simulink model "Kubon_lab10_3_sim"  (R2020b)
settings: Solver=VariableStepAuto  StartTime=0.0  StopTime=T_stop  RelTol=1e-3
values from neighbouring files (symbols this model uses):
  A = [ (-cpN*ppN*fk0-ks1-k0)/(Cv1) , k0/Cv1 ; (k0+cpN*ppN*fk0)/(Cv2) , (-k0-cpN*ppN*fk0-ks2)/(Cv2)  ]    [Kubon_lab10.m]    (also in Kubon_lab8.m = [-a1/A1 , a1/A1 ; a1/A2 , (-a1-a2)/A2])
  B = [(cpN*ppN*fk0)/(Cv1) , ks2/Cv1 ; 0 , ks2/Cv2 ]    [Kubon_lab10.m]    (also in Kubon_lab8.m = [1/A1 , 0 ; 0 , 1/A2])
  C = eye(2)    [Kubon_lab10.m]    (also in Kubon_lab8.m)
  D = zeros(2)    [Kubon_lab10.m]    (also in Kubon_lab8.m)
  dTkz = 2.0    (= 2)    [Kubon_lab10.m]    (also in Kubon_lab9.m = 0)
  dTzew = 0.0    (= 0)    [Kubon_lab10.m]    (also in Kubon_lab9.m)
  t0 = 50.0    (= 50)    [Kubon_lab10.m]    (also in Kubon_lab4.m = 5; Kubon_lab5.m = 0; Kubon_lab6.m = 5; Kubon_lab6_test.m = 0)
  Tkz0 = TkzN*0.7    (= 21)    [Kubon_lab10.m]    (also in Kubon_lab9.m = 30)
  Tw0_w = [Tw10,Tw20]    [Kubon_lab10.m]
  Tzew0 = TzewN    (= -20)    [Kubon_lab10.m]    (also in Kubon_lab9.m)
settings Model: Creator=pkubo  LastModifiedBy=pkubo

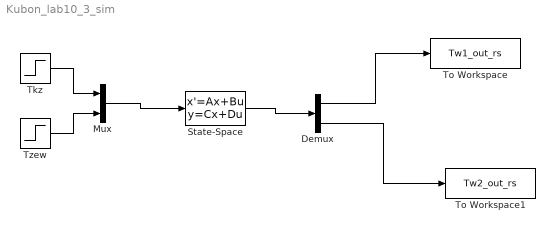
== system Kubon_lab10_3_sim ==
  Demux : Demux  Outputs=2
  Mux : Mux  Inputs=2
  State-Space : StateSpace  A=A  B=B  C=C  D=D  InitialCondition=Tw0_w
  Tkz : Step  Time=t0  Before=Tkz0  After=Tkz0+dTkz  SampleTime=0
  To Workspace : ToWorkspace  VariableName=Tw1_out_rs  SampleTime=-1
  To Workspace1 : ToWorkspace  VariableName=Tw2_out_rs  SampleTime=-1
  Tzew : Step  Time=t0  Before=Tzew0  After=Tzew0+dTzew  SampleTime=0
  wires:
  Demux/2 -> To Workspace1/1
  Tkz/1 -> Mux/1
  Demux/1 -> To Workspace/1
  State-Space/1 -> Demux/1
  Mux/1 -> State-Space/1
  Tzew/1 -> Mux/2
